simulink model "gm_FCS_MPC_3Phase_SPMSM_V1"  (R2022a)
settings: Solver=ode23t  StartTime=0.0  StopTime=0.2  RelTol=1e-3  AbsTol=1e-3  EnableMultiTasking=on
undefined symbols (not defined in the file or in its folder): f_c, Ld, Lq, np, psiPM, R, T_50MHz, u_dc
libraries: hdlmdlgenlib x28, dspsigops x26, ee_lib x22, nesl_utility x22, fl_lib x21, simulink x7
(part 5 of 5)

== system gm_FCS_MPC_3Phase_SPMSM_V1/Microcontroller Software/Subsystem1/MATLAB Function/multiplier72 ==
  In1 : Inport
  In2 : Inport  Port=2
  multiplier72 : Product  Inputs=**  OutDataTypeStr=single  SampleTime=1e-10
  multiplier72_pd1 : Delay  DelayLength=6
  Out1 : Outport
  wires:
  In1/1 -> multiplier72/1
  In2/1 -> multiplier72/2
  multiplier72/1 -> multiplier72_pd1/1
  multiplier72_pd1/1 -> Out1/1

== system gm_FCS_MPC_3Phase_SPMSM_V1/Microcontroller Software/Subsystem1/MATLAB Function/multiplier73 ==
  In1 : Inport
  In2 : Inport  Port=2
  multiplier73 : Product  Inputs=**  OutDataTypeStr=single  SampleTime=1e-10
  multiplier73_pd1 : Delay  DelayLength=6
  Out1 : Outport
  wires:
  In1/1 -> multiplier73/1
  In2/1 -> multiplier73/2
  multiplier73/1 -> multiplier73_pd1/1
  multiplier73_pd1/1 -> Out1/1

== system gm_FCS_MPC_3Phase_SPMSM_V1/Microcontroller Software/Subsystem1/MATLAB Function/multiplier74 ==
  In1 : Inport
  In2 : Inport  Port=2
  multiplier74 : Product  Inputs=**  OutDataTypeStr=single  SampleTime=1e-10
  multiplier74_pd1 : Delay  DelayLength=6
  Out1 : Outport
  wires:
  In1/1 -> multiplier74/1
  In2/1 -> multiplier74/2
  multiplier74/1 -> multiplier74_pd1/1
  multiplier74_pd1/1 -> Out1/1

== system gm_FCS_MPC_3Phase_SPMSM_V1/Microcontroller Software/Subsystem1/MATLAB Function/multiplier75 ==
  In1 : Inport
  In2 : Inport  Port=2
  multiplier75 : Product  Inputs=**  OutDataTypeStr=single  SampleTime=1e-10
  multiplier75_pd1 : Delay  DelayLength=6
  Out1 : Outport
  wires:
  In1/1 -> multiplier75/1
  In2/1 -> multiplier75/2
  multiplier75/1 -> multiplier75_pd1/1
  multiplier75_pd1/1 -> Out1/1

== system gm_FCS_MPC_3Phase_SPMSM_V1/Microcontroller Software/Subsystem1/MATLAB Function/multiplier76 ==
  In1 : Inport
  In2 : Inport  Port=2
  multiplier76 : Product  Inputs=**  OutDataTypeStr=single  SampleTime=1e-10
  multiplier76_pd1 : Delay  DelayLength=6
  Out1 : Outport
  wires:
  In1/1 -> multiplier76/1
  In2/1 -> multiplier76/2
  multiplier76/1 -> multiplier76_pd1/1
  multiplier76_pd1/1 -> Out1/1

== system gm_FCS_MPC_3Phase_SPMSM_V1/Microcontroller Software/Subsystem1/MATLAB Function/multiplier77 ==
  In1 : Inport
  In2 : Inport  Port=2
  multiplier77 : Product  Inputs=**  OutDataTypeStr=single  SampleTime=1e-10
  multiplier77_pd1 : Delay  DelayLength=6
  Out1 : Outport
  wires:
  In1/1 -> multiplier77/1
  In2/1 -> multiplier77/2
  multiplier77/1 -> multiplier77_pd1/1
  multiplier77_pd1/1 -> Out1/1

== system gm_FCS_MPC_3Phase_SPMSM_V1/Microcontroller Software/Subsystem1/MATLAB Function/multiplier78 ==
  In1 : Inport
  In2 : Inport  Port=2
  multiplier78 : Product  Inputs=**  OutDataTypeStr=single  SampleTime=1e-10
  multiplier78_pd1 : Delay  DelayLength=6
  Out1 : Outport
  wires:
  In1/1 -> multiplier78/1
  In2/1 -> multiplier78/2
  multiplier78/1 -> multiplier78_pd1/1
  multiplier78_pd1/1 -> Out1/1

== system gm_FCS_MPC_3Phase_SPMSM_V1/Microcontroller Software/Subsystem1/MATLAB Function/multiplier79 ==
  In1 : Inport
  In2 : Inport  Port=2
  multiplier79 : Product  Inputs=**  OutDataTypeStr=single  SampleTime=1e-10
  multiplier79_pd1 : Delay  DelayLength=6
  Out1 : Outport
  wires:
  In1/1 -> multiplier79/1
  In2/1 -> multiplier79/2
  multiplier79/1 -> multiplier79_pd1/1
  multiplier79_pd1/1 -> Out1/1

== system gm_FCS_MPC_3Phase_SPMSM_V1/Microcontroller Software/Subsystem1/MATLAB Function/multiplier8 ==
  In1 : Inport
  In2 : Inport  Port=2
  multiplier8 : Product  Inputs=**  OutDataTypeStr=single  SampleTime=1e-10
  multiplier8_pd1 : Delay  DelayLength=6
  Out1 : Outport
  wires:
  In1/1 -> multiplier8/1
  In2/1 -> multiplier8/2
  multiplier8/1 -> multiplier8_pd1/1
  multiplier8_pd1/1 -> Out1/1

== system gm_FCS_MPC_3Phase_SPMSM_V1/Microcontroller Software/Subsystem1/MATLAB Function/multiplier80 ==
  In1 : Inport
  In2 : Inport  Port=2
  multiplier80 : Product  Inputs=**  OutDataTypeStr=single  SampleTime=1e-10
  multiplier80_pd1 : Delay  DelayLength=6
  Out1 : Outport
  wires:
  In1/1 -> multiplier80/1
  In2/1 -> multiplier80/2
  multiplier80/1 -> multiplier80_pd1/1
  multiplier80_pd1/1 -> Out1/1

== system gm_FCS_MPC_3Phase_SPMSM_V1/Microcontroller Software/Subsystem1/MATLAB Function/multiplier81 ==
  In1 : Inport
  In2 : Inport  Port=2
  multiplier81 : Product  Inputs=**  OutDataTypeStr=single  SampleTime=1e-10
  multiplier81_pd1 : Delay  DelayLength=6
  Out1 : Outport
  wires:
  In1/1 -> multiplier81/1
  In2/1 -> multiplier81/2
  multiplier81/1 -> multiplier81_pd1/1
  multiplier81_pd1/1 -> Out1/1

== system gm_FCS_MPC_3Phase_SPMSM_V1/Microcontroller Software/Subsystem1/MATLAB Function/multiplier82 ==
  In1 : Inport
  In2 : Inport  Port=2
  multiplier82 : Product  Inputs=**  OutDataTypeStr=single  SampleTime=1e-10
  multiplier82_pd1 : Delay  DelayLength=6
  Out1 : Outport
  wires:
  In1/1 -> multiplier82/1
  In2/1 -> multiplier82/2
  multiplier82/1 -> multiplier82_pd1/1
  multiplier82_pd1/1 -> Out1/1

== system gm_FCS_MPC_3Phase_SPMSM_V1/Microcontroller Software/Subsystem1/MATLAB Function/multiplier83 ==
  In1 : Inport
  In2 : Inport  Port=2
  multiplier83 : Product  Inputs=**  OutDataTypeStr=single  SampleTime=1e-10
  multiplier83_pd1 : Delay  DelayLength=6
  Out1 : Outport
  wires:
  In1/1 -> multiplier83/1
  In2/1 -> multiplier83/2
  multiplier83/1 -> multiplier83_pd1/1
  multiplier83_pd1/1 -> Out1/1

== system gm_FCS_MPC_3Phase_SPMSM_V1/Microcontroller Software/Subsystem1/MATLAB Function/multiplier84 ==
  In1 : Inport
  In2 : Inport  Port=2
  multiplier84 : Product  Inputs=**  OutDataTypeStr=single  SampleTime=1e-10
  multiplier84_pd1 : Delay  DelayLength=6
  Out1 : Outport
  wires:
  In1/1 -> multiplier84/1
  In2/1 -> multiplier84/2
  multiplier84/1 -> multiplier84_pd1/1
  multiplier84_pd1/1 -> Out1/1

== system gm_FCS_MPC_3Phase_SPMSM_V1/Microcontroller Software/Subsystem1/MATLAB Function/multiplier85 ==
  In1 : Inport
  In2 : Inport  Port=2
  multiplier85 : Product  Inputs=**  OutDataTypeStr=single  SampleTime=1e-10
  multiplier85_pd1 : Delay  DelayLength=6
  Out1 : Outport
  wires:
  In1/1 -> multiplier85/1
  In2/1 -> multiplier85/2
  multiplier85/1 -> multiplier85_pd1/1
  multiplier85_pd1/1 -> Out1/1

== system gm_FCS_MPC_3Phase_SPMSM_V1/Microcontroller Software/Subsystem1/MATLAB Function/multiplier86 ==
  In1 : Inport
  In2 : Inport  Port=2
  multiplier86 : Product  Inputs=**  OutDataTypeStr=single  SampleTime=1e-10
  multiplier86_pd1 : Delay  DelayLength=6
  Out1 : Outport
  wires:
  In1/1 -> multiplier86/1
  In2/1 -> multiplier86/2
  multiplier86/1 -> multiplier86_pd1/1
  multiplier86_pd1/1 -> Out1/1

== system gm_FCS_MPC_3Phase_SPMSM_V1/Microcontroller Software/Subsystem1/MATLAB Function/multiplier87 ==
  In1 : Inport
  In2 : Inport  Port=2
  multiplier87 : Product  Inputs=**  OutDataTypeStr=single  SampleTime=1e-10
  multiplier87_pd1 : Delay  DelayLength=6
  Out1 : Outport
  wires:
  In1/1 -> multiplier87/1
  In2/1 -> multiplier87/2
  multiplier87/1 -> multiplier87_pd1/1
  multiplier87_pd1/1 -> Out1/1

== system gm_FCS_MPC_3Phase_SPMSM_V1/Microcontroller Software/Subsystem1/MATLAB Function/multiplier88 ==
  In1 : Inport
  In2 : Inport  Port=2
  multiplier88 : Product  Inputs=**  OutDataTypeStr=single  SampleTime=1e-10
  multiplier88_pd1 : Delay  DelayLength=6
  Out1 : Outport
  wires:
  In1/1 -> multiplier88/1
  In2/1 -> multiplier88/2
  multiplier88/1 -> multiplier88_pd1/1
  multiplier88_pd1/1 -> Out1/1

== system gm_FCS_MPC_3Phase_SPMSM_V1/Microcontroller Software/Subsystem1/MATLAB Function/multiplier89 ==
  In1 : Inport
  In2 : Inport  Port=2
  multiplier89 : Product  Inputs=**  OutDataTypeStr=single  SampleTime=1e-10
  multiplier89_pd1 : Delay  DelayLength=6
  Out1 : Outport
  wires:
  In1/1 -> multiplier89/1
  In2/1 -> multiplier89/2
  multiplier89/1 -> multiplier89_pd1/1
  multiplier89_pd1/1 -> Out1/1

== system gm_FCS_MPC_3Phase_SPMSM_V1/Microcontroller Software/Subsystem1/MATLAB Function/multiplier9 ==
  In1 : Inport
  In2 : Inport  Port=2
  multiplier9 : Product  Inputs=**  OutDataTypeStr=single  SampleTime=1e-10
  multiplier9_pd1 : Delay  DelayLength=6
  Out1 : Outport
  wires:
  In1/1 -> multiplier9/1
  In2/1 -> multiplier9/2
  multiplier9/1 -> multiplier9_pd1/1
  multiplier9_pd1/1 -> Out1/1

== system gm_FCS_MPC_3Phase_SPMSM_V1/Microcontroller Software/Subsystem1/MATLAB Function/multiplier90 ==
  In1 : Inport
  In2 : Inport  Port=2
  multiplier90 : Product  Inputs=**  OutDataTypeStr=single  SampleTime=1e-10
  multiplier90_pd1 : Delay  DelayLength=6
  Out1 : Outport
  wires:
  In1/1 -> multiplier90/1
  In2/1 -> multiplier90/2
  multiplier90/1 -> multiplier90_pd1/1
  multiplier90_pd1/1 -> Out1/1

== system gm_FCS_MPC_3Phase_SPMSM_V1/Microcontroller Software/Subsystem1/MATLAB Function/multiplier91 ==
  In1 : Inport
  In2 : Inport  Port=2
  multiplier91 : Product  Inputs=**  OutDataTypeStr=single  SampleTime=1e-10
  multiplier91_pd1 : Delay  DelayLength=6
  Out1 : Outport
  wires:
  In1/1 -> multiplier91/1
  In2/1 -> multiplier91/2
  multiplier91/1 -> multiplier91_pd1/1
  multiplier91_pd1/1 -> Out1/1

== system gm_FCS_MPC_3Phase_SPMSM_V1/Microcontroller Software/Subsystem1/MATLAB Function/multiplier92 ==
  In1 : Inport
  In2 : Inport  Port=2
  multiplier92 : Product  Inputs=**  OutDataTypeStr=single  SampleTime=1e-10
  multiplier92_pd1 : Delay  DelayLength=6
  Out1 : Outport
  wires:
  In1/1 -> multiplier92/1
  In2/1 -> multiplier92/2
  multiplier92/1 -> multiplier92_pd1/1
  multiplier92_pd1/1 -> Out1/1

== system gm_FCS_MPC_3Phase_SPMSM_V1/Microcontroller Software/Subsystem1/MATLAB Function/multiplier93 ==
  In1 : Inport
  In2 : Inport  Port=2
  multiplier93 : Product  Inputs=**  OutDataTypeStr=single  SampleTime=1e-10
  multiplier93_pd1 : Delay  DelayLength=6
  Out1 : Outport
  wires:
  In1/1 -> multiplier93/1
  In2/1 -> multiplier93/2
  multiplier93/1 -> multiplier93_pd1/1
  multiplier93_pd1/1 -> Out1/1

== system gm_FCS_MPC_3Phase_SPMSM_V1/Microcontroller Software/Subsystem1/MATLAB Function/multiplier94 ==
  In1 : Inport
  In2 : Inport  Port=2
  multiplier94 : Product  Inputs=**  OutDataTypeStr=single  SampleTime=1e-10
  multiplier94_pd1 : Delay  DelayLength=6
  Out1 : Outport
  wires:
  In1/1 -> multiplier94/1
  In2/1 -> multiplier94/2
  multiplier94/1 -> multiplier94_pd1/1
  multiplier94_pd1/1 -> Out1/1

== system gm_FCS_MPC_3Phase_SPMSM_V1/Microcontroller Software/Subsystem1/MATLAB Function/multiplier95 ==
  In1 : Inport
  In2 : Inport  Port=2
  multiplier95 : Product  Inputs=**  OutDataTypeStr=single  SampleTime=1e-10
  multiplier95_pd1 : Delay  DelayLength=6
  Out1 : Outport
  wires:
  In1/1 -> multiplier95/1
  In2/1 -> multiplier95/2
  multiplier95/1 -> multiplier95_pd1/1
  multiplier95_pd1/1 -> Out1/1

== system gm_FCS_MPC_3Phase_SPMSM_V1/Microcontroller Software/Subsystem1/MATLAB Function/multiplier96 ==
  In1 : Inport
  In2 : Inport  Port=2
  multiplier96 : Product  Inputs=**  OutDataTypeStr=single  SampleTime=1e-10
  multiplier96_pd1 : Delay  DelayLength=6
  Out1 : Outport
  wires:
  In1/1 -> multiplier96/1
  In2/1 -> multiplier96/2
  multiplier96/1 -> multiplier96_pd1/1
  multiplier96_pd1/1 -> Out1/1

== system gm_FCS_MPC_3Phase_SPMSM_V1/Microcontroller Software/Subsystem1/MATLAB Function/multiplier97 ==
  In1 : Inport
  In2 : Inport  Port=2
  multiplier97 : Product  Inputs=**  OutDataTypeStr=single  SampleTime=1e-10
  multiplier97_pd1 : Delay  DelayLength=6
  Out1 : Outport
  wires:
  In1/1 -> multiplier97/1
  In2/1 -> multiplier97/2
  multiplier97/1 -> multiplier97_pd1/1
  multiplier97_pd1/1 -> Out1/1

== system gm_FCS_MPC_3Phase_SPMSM_V1/Microcontroller Software/Subsystem1/MATLAB Function/multiplier98 ==
  In1 : Inport
  In2 : Inport  Port=2
  multiplier98 : Product  Inputs=**  OutDataTypeStr=single  SampleTime=1e-10
  multiplier98_pd1 : Delay  DelayLength=6
  Out1 : Outport
  wires:
  In1/1 -> multiplier98/1
  In2/1 -> multiplier98/2
  multiplier98/1 -> multiplier98_pd1/1
  multiplier98_pd1/1 -> Out1/1

== system gm_FCS_MPC_3Phase_SPMSM_V1/Microcontroller Software/Subsystem1/MATLAB Function/multiplier99 ==
  In1 : Inport
  In2 : Inport  Port=2
  multiplier99 : Product  Inputs=**  OutDataTypeStr=single  SampleTime=1e-10
  multiplier99_pd1 : Delay  DelayLength=6
  Out1 : Outport
  wires:
  In1/1 -> multiplier99/1
  In2/1 -> multiplier99/2
  multiplier99/1 -> multiplier99_pd1/1
  multiplier99_pd1/1 -> Out1/1

== system gm_FCS_MPC_3Phase_SPMSM_V1/Microcontroller Software/Subsystem1/MATLAB Function/square ==
  In1 : Inport
  In2 : Inport  Port=2
  square : Product  Inputs=**  OutDataTypeStr=single  SampleTime=1e-10
  square_pd1 : Delay  DelayLength=6
  Out1 : Outport
  wires:
  In1/1 -> square/1
  In2/1 -> square/2
  square/1 -> square_pd1/1
  square_pd1/1 -> Out1/1

== system gm_FCS_MPC_3Phase_SPMSM_V1/Microcontroller Software/Subsystem1/MATLAB Function/square1 ==
  In1 : Inport
  In2 : Inport  Port=2
  square1 : Product  Inputs=**  OutDataTypeStr=single  SampleTime=1e-10
  square1_pd1 : Delay  DelayLength=6
  Out1 : Outport
  wires:
  In1/1 -> square1/1
  In2/1 -> square1/2
  square1/1 -> square1_pd1/1
  square1_pd1/1 -> Out1/1

== system gm_FCS_MPC_3Phase_SPMSM_V1/Microcontroller Software/Subsystem1/MATLAB Function/square10 ==
  In1 : Inport
  In2 : Inport  Port=2
  square10 : Product  Inputs=**  OutDataTypeStr=single  SampleTime=1e-10
  square10_pd1 : Delay  DelayLength=6
  Out1 : Outport
  wires:
  In1/1 -> square10/1
  In2/1 -> square10/2
  square10/1 -> square10_pd1/1
  square10_pd1/1 -> Out1/1

== system gm_FCS_MPC_3Phase_SPMSM_V1/Microcontroller Software/Subsystem1/MATLAB Function/square11 ==
  In1 : Inport
  In2 : Inport  Port=2
  square11 : Product  Inputs=**  OutDataTypeStr=single  SampleTime=1e-10
  square11_pd1 : Delay  DelayLength=6
  Out1 : Outport
  wires:
  In1/1 -> square11/1
  In2/1 -> square11/2
  square11/1 -> square11_pd1/1
  square11_pd1/1 -> Out1/1

== system gm_FCS_MPC_3Phase_SPMSM_V1/Microcontroller Software/Subsystem1/MATLAB Function/square12 ==
  In1 : Inport
  In2 : Inport  Port=2
  square12 : Product  Inputs=**  OutDataTypeStr=single  SampleTime=1e-10
  square12_pd1 : Delay  DelayLength=6
  Out1 : Outport
  wires:
  In1/1 -> square12/1
  In2/1 -> square12/2
  square12/1 -> square12_pd1/1
  square12_pd1/1 -> Out1/1

== system gm_FCS_MPC_3Phase_SPMSM_V1/Microcontroller Software/Subsystem1/MATLAB Function/square13 ==
  In1 : Inport
  In2 : Inport  Port=2
  square13 : Product  Inputs=**  OutDataTypeStr=single  SampleTime=1e-10
  square13_pd1 : Delay  DelayLength=6
  Out1 : Outport
  wires:
  In1/1 -> square13/1
  In2/1 -> square13/2
  square13/1 -> square13_pd1/1
  square13_pd1/1 -> Out1/1

== system gm_FCS_MPC_3Phase_SPMSM_V1/Microcontroller Software/Subsystem1/MATLAB Function/square14 ==
  In1 : Inport
  In2 : Inport  Port=2
  square14 : Product  Inputs=**  OutDataTypeStr=single  SampleTime=1e-10
  square14_pd1 : Delay  DelayLength=6
  Out1 : Outport
  wires:
  In1/1 -> square14/1
  In2/1 -> square14/2
  square14/1 -> square14_pd1/1
  square14_pd1/1 -> Out1/1

== system gm_FCS_MPC_3Phase_SPMSM_V1/Microcontroller Software/Subsystem1/MATLAB Function/square15 ==
  In1 : Inport
  In2 : Inport  Port=2
  square15 : Product  Inputs=**  OutDataTypeStr=single  SampleTime=1e-10
  square15_pd1 : Delay  DelayLength=6
  Out1 : Outport
  wires:
  In1/1 -> square15/1
  In2/1 -> square15/2
  square15/1 -> square15_pd1/1
  square15_pd1/1 -> Out1/1

== system gm_FCS_MPC_3Phase_SPMSM_V1/Microcontroller Software/Subsystem1/MATLAB Function/square2 ==
  In1 : Inport
  In2 : Inport  Port=2
  square2 : Product  Inputs=**  OutDataTypeStr=single  SampleTime=1e-10
  square2_pd1 : Delay  DelayLength=6
  Out1 : Outport
  wires:
  In1/1 -> square2/1
  In2/1 -> square2/2
  square2/1 -> square2_pd1/1
  square2_pd1/1 -> Out1/1

== system gm_FCS_MPC_3Phase_SPMSM_V1/Microcontroller Software/Subsystem1/MATLAB Function/square3 ==
  In1 : Inport
  In2 : Inport  Port=2
  square3 : Product  Inputs=**  OutDataTypeStr=single  SampleTime=1e-10
  square3_pd1 : Delay  DelayLength=6
  Out1 : Outport
  wires:
  In1/1 -> square3/1
  In2/1 -> square3/2
  square3/1 -> square3_pd1/1
  square3_pd1/1 -> Out1/1

== system gm_FCS_MPC_3Phase_SPMSM_V1/Microcontroller Software/Subsystem1/MATLAB Function/square4 ==
  In1 : Inport
  In2 : Inport  Port=2
  square4 : Product  Inputs=**  OutDataTypeStr=single  SampleTime=1e-10
  square4_pd1 : Delay  DelayLength=6
  Out1 : Outport
  wires:
  In1/1 -> square4/1
  In2/1 -> square4/2
  square4/1 -> square4_pd1/1
  square4_pd1/1 -> Out1/1

== system gm_FCS_MPC_3Phase_SPMSM_V1/Microcontroller Software/Subsystem1/MATLAB Function/square5 ==
  In1 : Inport
  In2 : Inport  Port=2
  square5 : Product  Inputs=**  OutDataTypeStr=single  SampleTime=1e-10
  square5_pd1 : Delay  DelayLength=6
  Out1 : Outport
  wires:
  In1/1 -> square5/1
  In2/1 -> square5/2
  square5/1 -> square5_pd1/1
  square5_pd1/1 -> Out1/1

== system gm_FCS_MPC_3Phase_SPMSM_V1/Microcontroller Software/Subsystem1/MATLAB Function/square6 ==
  In1 : Inport
  In2 : Inport  Port=2
  square6 : Product  Inputs=**  OutDataTypeStr=single  SampleTime=1e-10
  square6_pd1 : Delay  DelayLength=6
  Out1 : Outport
  wires:
  In1/1 -> square6/1
  In2/1 -> square6/2
  square6/1 -> square6_pd1/1
  square6_pd1/1 -> Out1/1

== system gm_FCS_MPC_3Phase_SPMSM_V1/Microcontroller Software/Subsystem1/MATLAB Function/square7 ==
  In1 : Inport
  In2 : Inport  Port=2
  square7 : Product  Inputs=**  OutDataTypeStr=single  SampleTime=1e-10
  square7_pd1 : Delay  DelayLength=6
  Out1 : Outport
  wires:
  In1/1 -> square7/1
  In2/1 -> square7/2
  square7/1 -> square7_pd1/1
  square7_pd1/1 -> Out1/1

== system gm_FCS_MPC_3Phase_SPMSM_V1/Microcontroller Software/Subsystem1/MATLAB Function/square8 ==
  In1 : Inport
  In2 : Inport  Port=2
  square8 : Product  Inputs=**  OutDataTypeStr=single  SampleTime=1e-10
  square8_pd1 : Delay  DelayLength=6
  Out1 : Outport
  wires:
  In1/1 -> square8/1
  In2/1 -> square8/2
  square8/1 -> square8_pd1/1
  square8_pd1/1 -> Out1/1

== system gm_FCS_MPC_3Phase_SPMSM_V1/Microcontroller Software/Subsystem1/MATLAB Function/square9 ==
  In1 : Inport
  In2 : Inport  Port=2
  square9 : Product  Inputs=**  OutDataTypeStr=single  SampleTime=1e-10
  square9_pd1 : Delay  DelayLength=6
  Out1 : Outport
  wires:
  In1/1 -> square9/1
  In2/1 -> square9/2
  square9/1 -> square9_pd1/1
  square9_pd1/1 -> Out1/1

== system gm_FCS_MPC_3Phase_SPMSM_V1/Microcontroller Software/Subsystem1/MATLAB Function/subtract ==
  In1 : Inport
  In2 : Inport  Port=2
  subtract : Sum  Inputs=+-  OutDataTypeStr=single  SampleTime=1e-10
  subtract_pd1 : Delay  DelayLength=6
  Out1 : Outport
  wires:
  In1/1 -> subtract/1
  In2/1 -> subtract/2
  subtract/1 -> subtract_pd1/1
  subtract_pd1/1 -> Out1/1

== system gm_FCS_MPC_3Phase_SPMSM_V1/Microcontroller Software/Subsystem1/MATLAB Function/subtract1 ==
  In1 : Inport
  In2 : Inport  Port=2
  subtract1 : Sum  Inputs=+-  OutDataTypeStr=single  SampleTime=1e-10
  subtract1_pd1 : Delay  DelayLength=6
  Out1 : Outport
  wires:
  In1/1 -> subtract1/1
  In2/1 -> subtract1/2
  subtract1/1 -> subtract1_pd1/1
  subtract1_pd1/1 -> Out1/1

== system gm_FCS_MPC_3Phase_SPMSM_V1/Microcontroller Software/Subsystem1/MATLAB Function/subtract10 ==
  In1 : Inport
  In2 : Inport  Port=2
  subtract10 : Sum  Inputs=+-  OutDataTypeStr=single  SampleTime=1e-10
  subtract10_pd1 : Delay  DelayLength=6
  Out1 : Outport
  wires:
  In1/1 -> subtract10/1
  In2/1 -> subtract10/2
  subtract10/1 -> subtract10_pd1/1
  subtract10_pd1/1 -> Out1/1

== system gm_FCS_MPC_3Phase_SPMSM_V1/Microcontroller Software/Subsystem1/MATLAB Function/subtract11 ==
  In1 : Inport
  In2 : Inport  Port=2
  subtract11 : Sum  Inputs=+-  OutDataTypeStr=single  SampleTime=1e-10
  subtract11_pd1 : Delay  DelayLength=6
  Out1 : Outport
  wires:
  In1/1 -> subtract11/1
  In2/1 -> subtract11/2
  subtract11/1 -> subtract11_pd1/1
  subtract11_pd1/1 -> Out1/1

== system gm_FCS_MPC_3Phase_SPMSM_V1/Microcontroller Software/Subsystem1/MATLAB Function/subtract12 ==
  In1 : Inport
  In2 : Inport  Port=2
  subtract12 : Sum  Inputs=+-  OutDataTypeStr=single  SampleTime=1e-10
  subtract12_pd1 : Delay  DelayLength=6
  Out1 : Outport
  wires:
  In1/1 -> subtract12/1
  In2/1 -> subtract12/2
  subtract12/1 -> subtract12_pd1/1
  subtract12_pd1/1 -> Out1/1

== system gm_FCS_MPC_3Phase_SPMSM_V1/Microcontroller Software/Subsystem1/MATLAB Function/subtract13 ==
  In1 : Inport
  In2 : Inport  Port=2
  subtract13 : Sum  Inputs=+-  OutDataTypeStr=single  SampleTime=1e-10
  subtract13_pd1 : Delay  DelayLength=6
  Out1 : Outport
  wires:
  In1/1 -> subtract13/1
  In2/1 -> subtract13/2
  subtract13/1 -> subtract13_pd1/1
  subtract13_pd1/1 -> Out1/1

== system gm_FCS_MPC_3Phase_SPMSM_V1/Microcontroller Software/Subsystem1/MATLAB Function/subtract14 ==
  In1 : Inport
  In2 : Inport  Port=2
  subtract14 : Sum  Inputs=+-  OutDataTypeStr=single  SampleTime=1e-10
  subtract14_pd1 : Delay  DelayLength=6
  Out1 : Outport
  wires:
  In1/1 -> subtract14/1
  In2/1 -> subtract14/2
  subtract14/1 -> subtract14_pd1/1
  subtract14_pd1/1 -> Out1/1

== system gm_FCS_MPC_3Phase_SPMSM_V1/Microcontroller Software/Subsystem1/MATLAB Function/subtract15 ==
  In1 : Inport
  In2 : Inport  Port=2
  subtract15 : Sum  Inputs=+-  OutDataTypeStr=single  SampleTime=1e-10
  subtract15_pd1 : Delay  DelayLength=6
  Out1 : Outport
  wires:
  In1/1 -> subtract15/1
  In2/1 -> subtract15/2
  subtract15/1 -> subtract15_pd1/1
  subtract15_pd1/1 -> Out1/1

== system gm_FCS_MPC_3Phase_SPMSM_V1/Microcontroller Software/Subsystem1/MATLAB Function/subtract16 ==
  In1 : Inport
  In2 : Inport  Port=2
  subtract16 : Sum  Inputs=+-  OutDataTypeStr=single  SampleTime=1e-10
  subtract16_pd1 : Delay  DelayLength=6
  Out1 : Outport
  wires:
  In1/1 -> subtract16/1
  In2/1 -> subtract16/2
  subtract16/1 -> subtract16_pd1/1
  subtract16_pd1/1 -> Out1/1

== system gm_FCS_MPC_3Phase_SPMSM_V1/Microcontroller Software/Subsystem1/MATLAB Function/subtract17 ==
  In1 : Inport
  In2 : Inport  Port=2
  subtract17 : Sum  Inputs=+-  OutDataTypeStr=single  SampleTime=1e-10
  subtract17_pd1 : Delay  DelayLength=6
  Out1 : Outport
  wires:
  In1/1 -> subtract17/1
  In2/1 -> subtract17/2
  subtract17/1 -> subtract17_pd1/1
  subtract17_pd1/1 -> Out1/1

== system gm_FCS_MPC_3Phase_SPMSM_V1/Microcontroller Software/Subsystem1/MATLAB Function/subtract18 ==
  In1 : Inport
  In2 : Inport  Port=2
  subtract18 : Sum  Inputs=+-  OutDataTypeStr=single  SampleTime=1e-10
  subtract18_pd1 : Delay  DelayLength=6
  Out1 : Outport
  wires:
  In1/1 -> subtract18/1
  In2/1 -> subtract18/2
  subtract18/1 -> subtract18_pd1/1
  subtract18_pd1/1 -> Out1/1

== system gm_FCS_MPC_3Phase_SPMSM_V1/Microcontroller Software/Subsystem1/MATLAB Function/subtract19 ==
  In1 : Inport
  In2 : Inport  Port=2
  subtract19 : Sum  Inputs=+-  OutDataTypeStr=single  SampleTime=1e-10
  subtract19_pd1 : Delay  DelayLength=6
  Out1 : Outport
  wires:
  In1/1 -> subtract19/1
  In2/1 -> subtract19/2
  subtract19/1 -> subtract19_pd1/1
  subtract19_pd1/1 -> Out1/1

== system gm_FCS_MPC_3Phase_SPMSM_V1/Microcontroller Software/Subsystem1/MATLAB Function/subtract2 ==
  In1 : Inport
  In2 : Inport  Port=2
  subtract2 : Sum  Inputs=+-  OutDataTypeStr=single  SampleTime=1e-10
  subtract2_pd1 : Delay  DelayLength=6
  Out1 : Outport
  wires:
  In1/1 -> subtract2/1
  In2/1 -> subtract2/2
  subtract2/1 -> subtract2_pd1/1
  subtract2_pd1/1 -> Out1/1

== system gm_FCS_MPC_3Phase_SPMSM_V1/Microcontroller Software/Subsystem1/MATLAB Function/subtract20 ==
  In1 : Inport
  In2 : Inport  Port=2
  subtract20 : Sum  Inputs=+-  OutDataTypeStr=single  SampleTime=1e-10
  subtract20_pd1 : Delay  DelayLength=6
  Out1 : Outport
  wires:
  In1/1 -> subtract20/1
  In2/1 -> subtract20/2
  subtract20/1 -> subtract20_pd1/1
  subtract20_pd1/1 -> Out1/1

== system gm_FCS_MPC_3Phase_SPMSM_V1/Microcontroller Software/Subsystem1/MATLAB Function/subtract21 ==
  In1 : Inport
  In2 : Inport  Port=2
  subtract21 : Sum  Inputs=+-  OutDataTypeStr=single  SampleTime=1e-10
  subtract21_pd1 : Delay  DelayLength=6
  Out1 : Outport
  wires:
  In1/1 -> subtract21/1
  In2/1 -> subtract21/2
  subtract21/1 -> subtract21_pd1/1
  subtract21_pd1/1 -> Out1/1

== system gm_FCS_MPC_3Phase_SPMSM_V1/Microcontroller Software/Subsystem1/MATLAB Function/subtract22 ==
  In1 : Inport
  In2 : Inport  Port=2
  subtract22 : Sum  Inputs=+-  OutDataTypeStr=single  SampleTime=1e-10
  subtract22_pd1 : Delay  DelayLength=6
  Out1 : Outport
  wires:
  In1/1 -> subtract22/1
  In2/1 -> subtract22/2
  subtract22/1 -> subtract22_pd1/1
  subtract22_pd1/1 -> Out1/1

== system gm_FCS_MPC_3Phase_SPMSM_V1/Microcontroller Software/Subsystem1/MATLAB Function/subtract23 ==
  In1 : Inport
  In2 : Inport  Port=2
  subtract23 : Sum  Inputs=+-  OutDataTypeStr=single  SampleTime=1e-10
  subtract23_pd1 : Delay  DelayLength=6
  Out1 : Outport
  wires:
  In1/1 -> subtract23/1
  In2/1 -> subtract23/2
  subtract23/1 -> subtract23_pd1/1
  subtract23_pd1/1 -> Out1/1

== system gm_FCS_MPC_3Phase_SPMSM_V1/Microcontroller Software/Subsystem1/MATLAB Function/subtract24 ==
  In1 : Inport
  In2 : Inport  Port=2
  subtract24 : Sum  Inputs=+-  OutDataTypeStr=single  SampleTime=1e-10
  subtract24_pd1 : Delay  DelayLength=6
  Out1 : Outport
  wires:
  In1/1 -> subtract24/1
  In2/1 -> subtract24/2
  subtract24/1 -> subtract24_pd1/1
  subtract24_pd1/1 -> Out1/1

== system gm_FCS_MPC_3Phase_SPMSM_V1/Microcontroller Software/Subsystem1/MATLAB Function/subtract25 ==
  In1 : Inport
  In2 : Inport  Port=2
  subtract25 : Sum  Inputs=+-  OutDataTypeStr=single  SampleTime=1e-10
  subtract25_pd1 : Delay  DelayLength=6
  Out1 : Outport
  wires:
  In1/1 -> subtract25/1
  In2/1 -> subtract25/2
  subtract25/1 -> subtract25_pd1/1
  subtract25_pd1/1 -> Out1/1

== system gm_FCS_MPC_3Phase_SPMSM_V1/Microcontroller Software/Subsystem1/MATLAB Function/subtract26 ==
  In1 : Inport
  In2 : Inport  Port=2
  subtract26 : Sum  Inputs=+-  OutDataTypeStr=single  SampleTime=1e-10
  subtract26_pd1 : Delay  DelayLength=6
  Out1 : Outport
  wires:
  In1/1 -> subtract26/1
  In2/1 -> subtract26/2
  subtract26/1 -> subtract26_pd1/1
  subtract26_pd1/1 -> Out1/1

== system gm_FCS_MPC_3Phase_SPMSM_V1/Microcontroller Software/Subsystem1/MATLAB Function/subtract27 ==
  In1 : Inport
  In2 : Inport  Port=2
  subtract27 : Sum  Inputs=+-  OutDataTypeStr=single  SampleTime=1e-10
  subtract27_pd1 : Delay  DelayLength=6
  Out1 : Outport
  wires:
  In1/1 -> subtract27/1
  In2/1 -> subtract27/2
  subtract27/1 -> subtract27_pd1/1
  subtract27_pd1/1 -> Out1/1

== system gm_FCS_MPC_3Phase_SPMSM_V1/Microcontroller Software/Subsystem1/MATLAB Function/subtract28 ==
  In1 : Inport
  In2 : Inport  Port=2
  subtract28 : Sum  Inputs=+-  OutDataTypeStr=single  SampleTime=1e-10
  subtract28_pd1 : Delay  DelayLength=6
  Out1 : Outport
  wires:
  In1/1 -> subtract28/1
  In2/1 -> subtract28/2
  subtract28/1 -> subtract28_pd1/1
  subtract28_pd1/1 -> Out1/1

== system gm_FCS_MPC_3Phase_SPMSM_V1/Microcontroller Software/Subsystem1/MATLAB Function/subtract29 ==
  In1 : Inport
  In2 : Inport  Port=2
  subtract29 : Sum  Inputs=+-  OutDataTypeStr=single  SampleTime=1e-10
  subtract29_pd1 : Delay  DelayLength=6
  Out1 : Outport
  wires:
  In1/1 -> subtract29/1
  In2/1 -> subtract29/2
  subtract29/1 -> subtract29_pd1/1
  subtract29_pd1/1 -> Out1/1

== system gm_FCS_MPC_3Phase_SPMSM_V1/Microcontroller Software/Subsystem1/MATLAB Function/subtract3 ==
  In1 : Inport
  In2 : Inport  Port=2
  subtract3 : Sum  Inputs=+-  OutDataTypeStr=single  SampleTime=1e-10
  subtract3_pd1 : Delay  DelayLength=6
  Out1 : Outport
  wires:
  In1/1 -> subtract3/1
  In2/1 -> subtract3/2
  subtract3/1 -> subtract3_pd1/1
  subtract3_pd1/1 -> Out1/1

== system gm_FCS_MPC_3Phase_SPMSM_V1/Microcontroller Software/Subsystem1/MATLAB Function/subtract30 ==
  In1 : Inport
  In2 : Inport  Port=2
  subtract30 : Sum  Inputs=+-  OutDataTypeStr=single  SampleTime=1e-10
  subtract30_pd1 : Delay  DelayLength=6
  Out1 : Outport
  wires:
  In1/1 -> subtract30/1
  In2/1 -> subtract30/2
  subtract30/1 -> subtract30_pd1/1
  subtract30_pd1/1 -> Out1/1

== system gm_FCS_MPC_3Phase_SPMSM_V1/Microcontroller Software/Subsystem1/MATLAB Function/subtract31 ==
  In1 : Inport
  In2 : Inport  Port=2
  subtract31 : Sum  Inputs=+-  OutDataTypeStr=single  SampleTime=1e-10
  subtract31_pd1 : Delay  DelayLength=6
  Out1 : Outport
  wires:
  In1/1 -> subtract31/1
  In2/1 -> subtract31/2
  subtract31/1 -> subtract31_pd1/1
  subtract31_pd1/1 -> Out1/1

== system gm_FCS_MPC_3Phase_SPMSM_V1/Microcontroller Software/Subsystem1/MATLAB Function/subtract32 ==
  In1 : Inport
  In2 : Inport  Port=2
  subtract32 : Sum  Inputs=+-  OutDataTypeStr=single  SampleTime=1e-10
  subtract32_pd1 : Delay  DelayLength=6
  Out1 : Outport
  wires:
  In1/1 -> subtract32/1
  In2/1 -> subtract32/2
  subtract32/1 -> subtract32_pd1/1
  subtract32_pd1/1 -> Out1/1

== system gm_FCS_MPC_3Phase_SPMSM_V1/Microcontroller Software/Subsystem1/MATLAB Function/subtract33 ==
  In1 : Inport
  In2 : Inport  Port=2
  subtract33 : Sum  Inputs=+-  OutDataTypeStr=single  SampleTime=1e-10
  subtract33_pd1 : Delay  DelayLength=6
  Out1 : Outport
  wires:
  In1/1 -> subtract33/1
  In2/1 -> subtract33/2
  subtract33/1 -> subtract33_pd1/1
  subtract33_pd1/1 -> Out1/1

== system gm_FCS_MPC_3Phase_SPMSM_V1/Microcontroller Software/Subsystem1/MATLAB Function/subtract34 ==
  In1 : Inport
  In2 : Inport  Port=2
  subtract34 : Sum  Inputs=+-  OutDataTypeStr=single  SampleTime=1e-10
  subtract34_pd1 : Delay  DelayLength=6
  Out1 : Outport
  wires:
  In1/1 -> subtract34/1
  In2/1 -> subtract34/2
  subtract34/1 -> subtract34_pd1/1
  subtract34_pd1/1 -> Out1/1

== system gm_FCS_MPC_3Phase_SPMSM_V1/Microcontroller Software/Subsystem1/MATLAB Function/subtract35 ==
  In1 : Inport
  In2 : Inport  Port=2
  subtract35 : Sum  Inputs=+-  OutDataTypeStr=single  SampleTime=1e-10
  subtract35_pd1 : Delay  DelayLength=6
  Out1 : Outport
  wires:
  In1/1 -> subtract35/1
  In2/1 -> subtract35/2
  subtract35/1 -> subtract35_pd1/1
  subtract35_pd1/1 -> Out1/1

== system gm_FCS_MPC_3Phase_SPMSM_V1/Microcontroller Software/Subsystem1/MATLAB Function/subtract36 ==
  In1 : Inport
  In2 : Inport  Port=2
  subtract36 : Sum  Inputs=+-  OutDataTypeStr=single  SampleTime=1e-10
  subtract36_pd1 : Delay  DelayLength=6
  Out1 : Outport
  wires:
  In1/1 -> subtract36/1
  In2/1 -> subtract36/2
  subtract36/1 -> subtract36_pd1/1
  subtract36_pd1/1 -> Out1/1

== system gm_FCS_MPC_3Phase_SPMSM_V1/Microcontroller Software/Subsystem1/MATLAB Function/subtract37 ==
  In1 : Inport
  In2 : Inport  Port=2
  subtract37 : Sum  Inputs=+-  OutDataTypeStr=single  SampleTime=1e-10
  subtract37_pd1 : Delay  DelayLength=6
  Out1 : Outport
  wires:
  In1/1 -> subtract37/1
  In2/1 -> subtract37/2
  subtract37/1 -> subtract37_pd1/1
  subtract37_pd1/1 -> Out1/1

== system gm_FCS_MPC_3Phase_SPMSM_V1/Microcontroller Software/Subsystem1/MATLAB Function/subtract38 ==
  In1 : Inport
  In2 : Inport  Port=2
  subtract38 : Sum  Inputs=+-  OutDataTypeStr=single  SampleTime=1e-10
  subtract38_pd1 : Delay  DelayLength=6
  Out1 : Outport
  wires:
  In1/1 -> subtract38/1
  In2/1 -> subtract38/2
  subtract38/1 -> subtract38_pd1/1
  subtract38_pd1/1 -> Out1/1

== system gm_FCS_MPC_3Phase_SPMSM_V1/Microcontroller Software/Subsystem1/MATLAB Function/subtract39 ==
  In1 : Inport
  In2 : Inport  Port=2
  subtract39 : Sum  Inputs=+-  OutDataTypeStr=single  SampleTime=1e-10
  subtract39_pd1 : Delay  DelayLength=6
  Out1 : Outport
  wires:
  In1/1 -> subtract39/1
  In2/1 -> subtract39/2
  subtract39/1 -> subtract39_pd1/1
  subtract39_pd1/1 -> Out1/1

== system gm_FCS_MPC_3Phase_SPMSM_V1/Microcontroller Software/Subsystem1/MATLAB Function/subtract4 ==
  In1 : Inport
  In2 : Inport  Port=2
  subtract4 : Sum  Inputs=+-  OutDataTypeStr=single  SampleTime=1e-10
  subtract4_pd1 : Delay  DelayLength=6
  Out1 : Outport
  wires:
  In1/1 -> subtract4/1
  In2/1 -> subtract4/2
  subtract4/1 -> subtract4_pd1/1
  subtract4_pd1/1 -> Out1/1

== system gm_FCS_MPC_3Phase_SPMSM_V1/Microcontroller Software/Subsystem1/MATLAB Function/subtract40 ==
  In1 : Inport
  In2 : Inport  Port=2
  subtract40 : Sum  Inputs=+-  OutDataTypeStr=single  SampleTime=1e-10
  subtract40_pd1 : Delay  DelayLength=6
  Out1 : Outport
  wires:
  In1/1 -> subtract40/1
  In2/1 -> subtract40/2
  subtract40/1 -> subtract40_pd1/1
  subtract40_pd1/1 -> Out1/1

== system gm_FCS_MPC_3Phase_SPMSM_V1/Microcontroller Software/Subsystem1/MATLAB Function/subtract41 ==
  In1 : Inport
  In2 : Inport  Port=2
  subtract41 : Sum  Inputs=+-  OutDataTypeStr=single  SampleTime=1e-10
  subtract41_pd1 : Delay  DelayLength=6
  Out1 : Outport
  wires:
  In1/1 -> subtract41/1
  In2/1 -> subtract41/2
  subtract41/1 -> subtract41_pd1/1
  subtract41_pd1/1 -> Out1/1

== system gm_FCS_MPC_3Phase_SPMSM_V1/Microcontroller Software/Subsystem1/MATLAB Function/subtract42 ==
  In1 : Inport
  In2 : Inport  Port=2
  subtract42 : Sum  Inputs=+-  OutDataTypeStr=single  SampleTime=1e-10
  subtract42_pd1 : Delay  DelayLength=6
  Out1 : Outport
  wires:
  In1/1 -> subtract42/1
  In2/1 -> subtract42/2
  subtract42/1 -> subtract42_pd1/1
  subtract42_pd1/1 -> Out1/1

== system gm_FCS_MPC_3Phase_SPMSM_V1/Microcontroller Software/Subsystem1/MATLAB Function/subtract5 ==
  In1 : Inport
  In2 : Inport  Port=2
  subtract5 : Sum  Inputs=+-  OutDataTypeStr=single  SampleTime=1e-10
  subtract5_pd1 : Delay  DelayLength=6
  Out1 : Outport
  wires:
  In1/1 -> subtract5/1
  In2/1 -> subtract5/2
  subtract5/1 -> subtract5_pd1/1
  subtract5_pd1/1 -> Out1/1

== system gm_FCS_MPC_3Phase_SPMSM_V1/Microcontroller Software/Subsystem1/MATLAB Function/subtract6 ==
  In1 : Inport
  In2 : Inport  Port=2
  subtract6 : Sum  Inputs=+-  OutDataTypeStr=single  SampleTime=1e-10
  subtract6_pd1 : Delay  DelayLength=6
  Out1 : Outport
  wires:
  In1/1 -> subtract6/1
  In2/1 -> subtract6/2
  subtract6/1 -> subtract6_pd1/1
  subtract6_pd1/1 -> Out1/1

== system gm_FCS_MPC_3Phase_SPMSM_V1/Microcontroller Software/Subsystem1/MATLAB Function/subtract7 ==
  In1 : Inport
  In2 : Inport  Port=2
  subtract7 : Sum  Inputs=+-  OutDataTypeStr=single  SampleTime=1e-10
  subtract7_pd1 : Delay  DelayLength=6
  Out1 : Outport
  wires:
  In1/1 -> subtract7/1
  In2/1 -> subtract7/2
  subtract7/1 -> subtract7_pd1/1
  subtract7_pd1/1 -> Out1/1

== system gm_FCS_MPC_3Phase_SPMSM_V1/Microcontroller Software/Subsystem1/MATLAB Function/subtract8 ==
  In1 : Inport
  In2 : Inport  Port=2
  subtract8 : Sum  Inputs=+-  OutDataTypeStr=single  SampleTime=1e-10
  subtract8_pd1 : Delay  DelayLength=6
  Out1 : Outport
  wires:
  In1/1 -> subtract8/1
  In2/1 -> subtract8/2
  subtract8/1 -> subtract8_pd1/1
  subtract8_pd1/1 -> Out1/1

== system gm_FCS_MPC_3Phase_SPMSM_V1/Microcontroller Software/Subsystem1/MATLAB Function/subtract9 ==
  In1 : Inport
  In2 : Inport  Port=2
  subtract9 : Sum  Inputs=+-  OutDataTypeStr=single  SampleTime=1e-10
  subtract9_pd1 : Delay  DelayLength=6
  Out1 : Outport
  wires:
  In1/1 -> subtract9/1
  In2/1 -> subtract9/2
  subtract9/1 -> subtract9_pd1/1
  subtract9_pd1/1 -> Out1/1

== system gm_FCS_MPC_3Phase_SPMSM_V1/Microcontroller Software/Subsystem1/MATLAB Function1/relop ==
  In1 : Inport
  In2 : Inport  Port=2
  relop : RelationalOperator  Operator=<  OutDataTypeStr=boolean  SampleTime=1e-10  InputSameDT=off
  relop_pd1 : Delay  DelayLength=1
  Out1 : Outport
  wires:
  In1/1 -> relop/1
  In2/1 -> relop/2
  relop/1 -> relop_pd1/1
  relop_pd1/1 -> Out1/1

== system gm_FCS_MPC_3Phase_SPMSM_V1/Microcontroller Software/Subsystem1/MATLAB Function1/relop1 ==
  In1 : Inport
  In2 : Inport  Port=2
  relop1 : RelationalOperator  Operator=<  OutDataTypeStr=boolean  SampleTime=1e-10  InputSameDT=off
  relop1_pd1 : Delay  DelayLength=1
  Out1 : Outport
  wires:
  In1/1 -> relop1/1
  In2/1 -> relop1/2
  relop1/1 -> relop1_pd1/1
  relop1_pd1/1 -> Out1/1

== system gm_FCS_MPC_3Phase_SPMSM_V1/Microcontroller Software/Subsystem1/MATLAB Function1/relop2 ==
  In1 : Inport
  In2 : Inport  Port=2
  relop2 : RelationalOperator  Operator=<  OutDataTypeStr=boolean  SampleTime=1e-10  InputSameDT=off
  relop2_pd1 : Delay  DelayLength=1
  Out1 : Outport
  wires:
  In1/1 -> relop2/1
  In2/1 -> relop2/2
  relop2/1 -> relop2_pd1/1
  relop2_pd1/1 -> Out1/1

== system gm_FCS_MPC_3Phase_SPMSM_V1/Microcontroller Software/Subsystem1/MATLAB Function1/relop3 ==
  In1 : Inport
  In2 : Inport  Port=2
  relop3 : RelationalOperator  Operator=<  OutDataTypeStr=boolean  SampleTime=1e-10  InputSameDT=off
  relop3_pd1 : Delay  DelayLength=1
  Out1 : Outport
  wires:
  In1/1 -> relop3/1
  In2/1 -> relop3/2
  relop3/1 -> relop3_pd1/1
  relop3_pd1/1 -> Out1/1

== system gm_FCS_MPC_3Phase_SPMSM_V1/Microcontroller Software/Subsystem1/MATLAB Function1/relop4 ==
  In1 : Inport
  In2 : Inport  Port=2
  relop4 : RelationalOperator  Operator=<  OutDataTypeStr=boolean  SampleTime=1e-10  InputSameDT=off
  relop4_pd1 : Delay  DelayLength=1
  Out1 : Outport
  wires:
  In1/1 -> relop4/1
  In2/1 -> relop4/2
  relop4/1 -> relop4_pd1/1
  relop4_pd1/1 -> Out1/1

== system gm_FCS_MPC_3Phase_SPMSM_V1/Microcontroller Software/Subsystem1/MATLAB Function1/relop5 ==
  In1 : Inport
  In2 : Inport  Port=2
  relop5 : RelationalOperator  Operator=<  OutDataTypeStr=boolean  SampleTime=1e-10  InputSameDT=off
  relop5_pd1 : Delay  DelayLength=1
  Out1 : Outport
  wires:
  In1/1 -> relop5/1
  In2/1 -> relop5/2
  relop5/1 -> relop5_pd1/1
  relop5_pd1/1 -> Out1/1

== system gm_FCS_MPC_3Phase_SPMSM_V1/Microcontroller Software/Subsystem1/MATLAB Function1/relop6 ==
  In1 : Inport
  In2 : Inport  Port=2
  relop6 : RelationalOperator  Operator=<  OutDataTypeStr=boolean  SampleTime=1e-10  InputSameDT=off
  relop6_pd1 : Delay  DelayLength=1
  Out1 : Outport
  wires:
  In1/1 -> relop6/1
  In2/1 -> relop6/2
  relop6/1 -> relop6_pd1/1
  relop6_pd1/1 -> Out1/1

== matlab function gm_FCS_MPC_3Phase_SPMSM_V1/3ph_Inverter/12bit ADC ==
  data: u input; y output
function y = fcn(u)
%#codegen

y = u*4095/3.3;

== matlab function gm_FCS_MPC_3Phase_SPMSM_V1/3ph_Inverter/12bit ADC1 ==
  data: u input; y output
function y = fcn(u)
%#codegen

y = u*4095/3.3;

== matlab function gm_FCS_MPC_3Phase_SPMSM_V1/3ph_Inverter/12bit ADC2 ==
  data: u input; y output
function y = fcn(u)
%#codegen

y = u*4095/3.3;

== matlab function gm_FCS_MPC_3Phase_SPMSM_V1/Microcontroller Software/Subsystem/MATLAB Function ==
  data: I input; Naechste_Schaltstellung output
function Naechste_Schaltstellung = fcn(I)

% Mögliche Schaltstellungen des Umrichters
Moegliche_Schaltstellungen=[0 1 0 1 0 1;1 0 0 1 0 1;1 0 1 0 0 1;0 1 1 0 0 1;0  1 1 0 1 0;0 1 0 1 1 0;1 0 0 1 1 0;1 0 1 0 1 0];

if I==0
    I=1;
end

% Ausgegebene Schaltstellung
Naechste_Schaltstellung=(Moegliche_Schaltstellungen(I,:))';

end
